simulink model "rollDynamicsLinear"  (R2017a)
settings: Solver=ode3  StartTime=0.0  StopTime=10  FixedStep=0.021  RelTol=1e-3  EnableMultiTasking=on
values from neighbouring files (symbols this model uses):
  enableMisErr = 1    [RollDynamics.m]    (also in RollDynamicsPWM-Theta.m = -1; rollDynamics.m)
  enableOutputPert = -1    [RollDynamics.m]    (also in RollDynamicsPWM-Theta.m)
  lambdaErr = 0.00001    (= 1e-05)    [RollDynamicsPWM-Theta.m]
  Mde = 70    [RollDynamicsPWM-Theta.m]
  Me = 15    [RollDynamicsPWM-Theta.m]
  roll_lin_den_84 = roll_lin_den_84{1,1}    [RollDynamicsPWM-Theta.m]
  roll_lin_num_84 = roll_lin_num_84{1,1}    [RollDynamicsPWM-Theta.m]
  Ts = 0.021    [RollDynamics.m]    (also in RollDynamicsPWM-Theta.m; rollDynamics.m)
undefined symbols (not defined in the file or in its folder): sigbuilder_block
libraries: simulink x7
settings Model: Creator=root  LastModifiedBy=userk
settings DataIOCC: LimitDataPoints=on  SaveFormat=Array
settings OptimizationCC: LifeSpan=inf
settings DebuggingCC: SolverPrmCheckMsg=warning  SFUnexpectedBacktrackingDiag=warning  SFNoUnconditionalDefaultTransitionDiag=warning  SFExecutionAtInitializationDiag=none
settings HardwareCC: ProdBitPerPointer=32  ProdBitPerSizeT=32  ProdBitPerPtrDiffT=32  ProdLargestAtomicFloat=None  ProdIntDivRoundTo=Undefined  ProdEndianess=Unspecified  ProdWordSize=32  ProdHWDeviceType=32-bit Generic
settings ModelReferenceCC: PropagateSignalLabelsOutOfModel=off
settings GRTTargetCC: TargetLangStandard=C89/C90 (ANSI)  GeneratePreprocessorConditionals=Disable all
settings ConfigComp: CovMetricSettings=dw  CovHtmlReporting=on  CovSaveCumulativeToWorkspaceVar=on  CovSaveSingleToWorkspaceVar=on  CovExternalEMLEnable=off  CovSFcnEnable=off

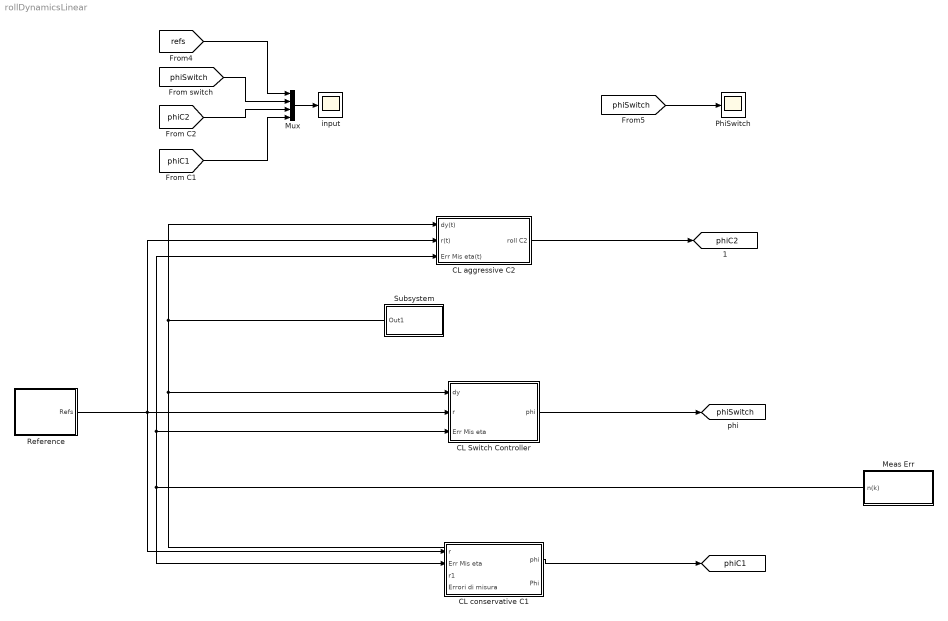
== system rollDynamicsLinear ==
  CL Switch Controller : Subsystem
  "CL aggressive C2 " : Subsystem
  CL conservative C1 : Subsystem
  Meas Err : Subsystem
  Mux : Mux
  PhiSwitch : Scope
  Reference : Subsystem
  Subsystem : Subsystem
  input : Scope
  tag scope: phiC1=global, phiC2=global, phiSwitch=global
  wires:
  Mux/1 -> input/1
  "CL aggressive C2 "/1(roll C2) -> [phiC2]
  CL conservative C1/1(phi) -> [phiC1]
  Reference/1(Refs) -> "CL aggressive C2 "/2(r(t)), CL Switch Controller/2(r), CL conservative C1/1(r)
  Subsystem/1(Out1) -> CL Switch Controller/1(dy), "CL aggressive C2 "/1(dy(t))
  Meas Err/1(n(k)) -> CL conservative C1/2(Err Mis eta), CL Switch Controller/3(Err Mis eta), "CL aggressive C2 "/3(Err Mis eta(t))
  CL Switch Controller/1(phi) -> [phiSwitch]
  [phiSwitch] -> Mux/2
  [phiC1] -> Mux/4
  [refs] -> Mux/1
  [phiSwitch] -> PhiSwitch/1
  [phiC2] -> Mux/3

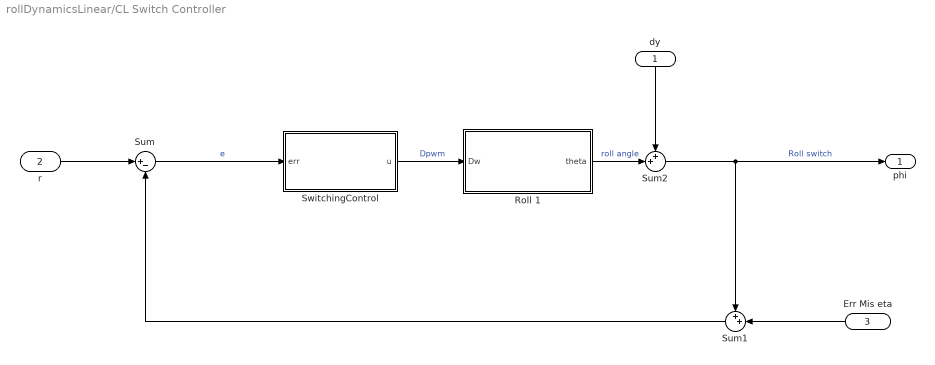
== system rollDynamicsLinear/CL Switch Controller ==
  dy : Inport
  r : Inport  Port=2
  Err Mis eta : Inport  Port=3
  Roll 1 : Subsystem
  Sum : Sum  Inputs=|+-
  Sum1 : Sum  Inputs=++|
  Sum2 : Sum  Inputs=++|
  "SwitchingControl " : Subsystem
  phi : Outport
  wires:
  r/1 -> Sum/1
  Sum2/1 -> phi/1, Sum1/1  "Roll switch"
  Roll 1/1("theta ") -> Sum2/2  "roll angle"
  "SwitchingControl "/1("u ") -> Roll 1/1("Dw ")  "Dpwm"
  Sum/1 -> "SwitchingControl "/1("err ")  "e"
  dy/1 -> Sum2/1
  Err Mis eta/1 -> Sum1/2
  Sum1/1 -> Sum/2

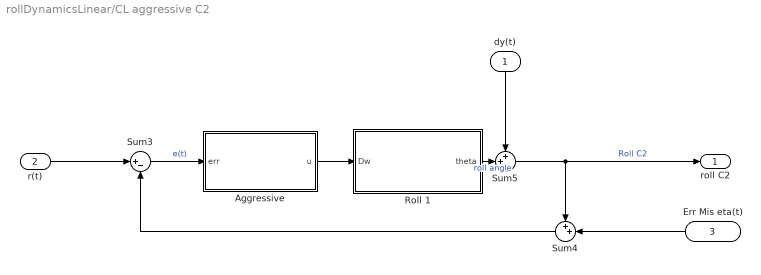
== system rollDynamicsLinear/CL aggressive C2  ==
  dy(t) : Inport
  r(t) : Inport  Port=2
  Err Mis eta(t) : Inport  Port=3
  "Aggressive " : Subsystem
  Roll 1 : Subsystem
  Sum3 : Sum  Inputs=|+-
  Sum4 : Sum  Inputs=++|
  Sum5 : Sum  Inputs=++|
  roll C2 : Outport
  wires:
  dy(t)/1 -> Sum5/1
  Sum3/1 -> "Aggressive "/1("err ")  "e(t)"
  "Aggressive "/1("u ") -> Roll 1/1("Dw ")
  Sum4/1 -> Sum3/2
  Sum5/1 -> roll C2/1, Sum4/1  "Roll C2"
  r(t)/1 -> Sum3/1
  Roll 1/1("theta ") -> Sum5/2  "roll angle"
  Err Mis eta(t)/1 -> Sum4/2

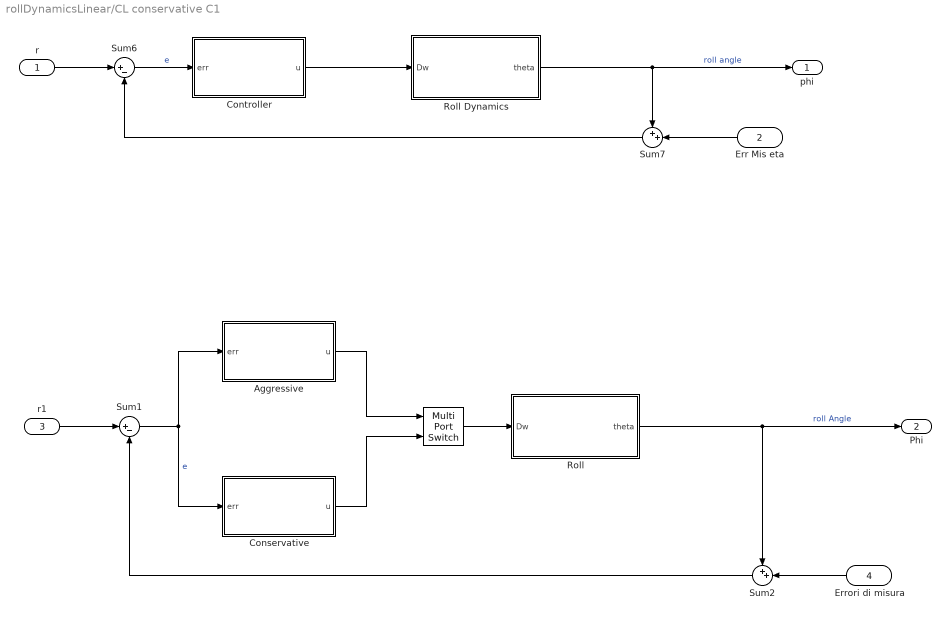
== system rollDynamicsLinear/CL conservative C1 ==
  r : Inport
  Err Mis eta : Inport  Port=2
  r1 : Inport  Port=3
  Errori di misura : Inport  Port=4
  " " : MultiPortSwitch  DataPortOrder=Zero-based contiguous  Inputs=1  zeroidx=on
  "Aggressive " : Subsystem
  Conservative : Subsystem
  Controller : Subsystem
  "Roll " : Subsystem
  "Roll Dynamics " : Subsystem
  Sum1 : Sum  Inputs=|+-
  Sum2 : Sum  Inputs=++|
  Sum6 : Sum  Inputs=|+-
  Sum7 : Sum  Inputs=++|
  phi : Outport
  Phi : Outport  Port=2
  wires:
  Err Mis eta/1 -> Sum7/2
  r/1 -> Sum6/1
  "Roll Dynamics "/1("theta ") -> phi/1, Sum7/1  "roll angle"
  Sum6/1 -> Controller/1("err ")  "e"
  Sum7/1 -> Sum6/2
  Controller/1("u ") -> "Roll Dynamics "/1("Dw ")
  Errori di misura/1 -> Sum2/2
  "Roll "/1("theta ") -> Phi/1, Sum2/1  "roll Angle"
  Sum1/1 -> Conservative/1("err "), "Aggressive "/1("err ")  "e"
  Sum2/1 -> Sum1/2
  r1/1 -> Sum1/1
  Conservative/1("u ") -> " "/2
  " "/1 -> "Roll "/1("Dw ")
  "Aggressive "/1("u ") -> " "/1

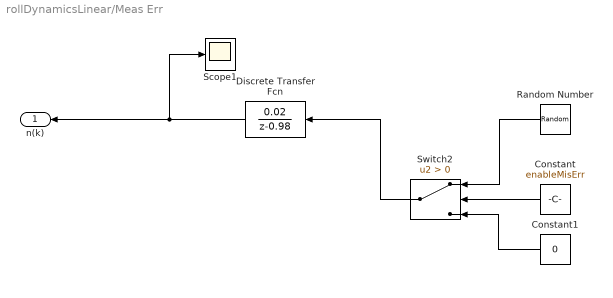
== system rollDynamicsLinear/Meas Err ==
  Constant : Constant  Value=enableMisErr
  Constant1 : Constant  Value=0
  Discrete Transfer Fcn : DiscreteTransferFcn  Numerator=[0.02]  Denominator=[1 -0.98]
  Random Number : RandomNumber  Variance=1.3  SampleTime=Ts
  Scope1 : Scope
  Switch2 : Switch  Criteria=u2 > Threshold  SampleTime=Ts
  n(k) : Outport
  wires:
  Constant1/1 -> Switch2/3
  Constant/1 -> Switch2/2
  Random Number/1 -> Switch2/1
  Switch2/1 -> Discrete Transfer Fcn/1
  Discrete Transfer Fcn/1 -> Scope1/1, n(k)/1

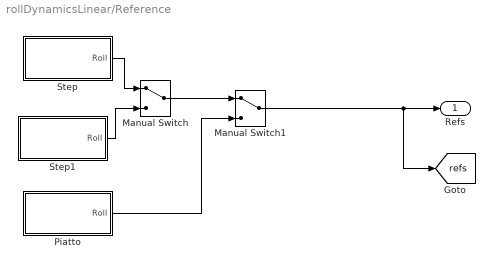
== system rollDynamicsLinear/Reference ==
  Manual Switch : ManualSwitch
  Manual Switch1 : ManualSwitch
  Piatto : Subsystem  Tag=STV Subsys  LoadFcn=sigbuilder_block('load');  StartFcn=sigbuilder_block('start');  StopFcn=sigbuilder_block('stop');  ClipboardFcn=sigbuilder_block('clipboard');  mask(Sigbuilder block){tuvar=[0:10]}
      mask help: Simulink:masks:SigbuilderBlock_MD
      mask init:
      | if ~strcmp(get_param(bdroot(gcbh),'SimulationStatus'),'stopped') tuvar = sigbuilder_block('maskInit'); end
      settings: CopyFcn=sigbuilder_block('copy');  DeleteFcn=sigbuilder_block('delete');  ModelCloseFcn=sigbuilder_block('modelClose');  PreSaveFcn=sigbuilder_block('preSave');  PauseFcn=sigbuilder_block('pause');  ContinueFcn=sigbuilder_block('continue');  NameChangeFcn=sigbuilder_block('namechange');  OpenFcn=sigbuilder_block('open',[240 0.75 594.75 533.25 ]);  CloseFcn=sigbuilder_block('close');
      mask Display: plot(0, 0, 100, 100,[2, 2, 32, 32, 2], [68, 8, 8, 68, 68],[32, 2], [38, 38], [32, 19, 2],[53, 60, 44], [32, 17, 17, 2],[16, 16, 31, 31]);txt = getActiveGroup(gcbh);text(2, 100, txt,'verticalAlignment', 'top');
  Step : Subsystem  Tag=STV Subsys  LoadFcn=sigbuilder_block('load');  StartFcn=sigbuilder_block('start');  StopFcn=sigbuilder_block('stop');  ClipboardFcn=sigbuilder_block('clipboard');  mask(Sigbuilder block){tuvar=[0:10]}
      mask help: Simulink:masks:SigbuilderBlock_MD
      mask init:
      | if ~strcmp(get_param(bdroot(gcbh),'SimulationStatus'),'stopped') tuvar = sigbuilder_block('maskInit'); end
      settings: CopyFcn=sigbuilder_block('copy');  DeleteFcn=sigbuilder_block('delete');  ModelCloseFcn=sigbuilder_block('modelClose');  PreSaveFcn=sigbuilder_block('preSave');  PauseFcn=sigbuilder_block('pause');  ContinueFcn=sigbuilder_block('continue');  NameChangeFcn=sigbuilder_block('namechange');  OpenFcn=sigbuilder_block('open',[222.75 0 632.25 495.75 ]);  CloseFcn=sigbuilder_block('close');
      mask Display: plot(0, 0, 100, 100,[2, 2, 32, 32, 2], [68, 8, 8, 68, 68],[32, 2], [38, 38], [32, 19, 2],[53, 60, 44], [32, 17, 17, 2],[16, 16, 31, 31]);txt = getActiveGroup(gcbh);text(2, 100, txt,'verticalAlignment', 'top');
  Step1 : Subsystem  Tag=STV Subsys  LoadFcn=sigbuilder_block('load');  StartFcn=sigbuilder_block('start');  StopFcn=sigbuilder_block('stop');  ClipboardFcn=sigbuilder_block('clipboard');  mask(Sigbuilder block){tuvar=[0:10]}
      mask help: Simulink:masks:SigbuilderBlock_MD
      mask init:
      | if ~strcmp(get_param(bdroot(gcbh),'SimulationStatus'),'stopped') tuvar = sigbuilder_block('maskInit'); end
      settings: CopyFcn=sigbuilder_block('copy');  DeleteFcn=sigbuilder_block('delete');  ModelCloseFcn=sigbuilder_block('modelClose');  PreSaveFcn=sigbuilder_block('preSave');  PauseFcn=sigbuilder_block('pause');  ContinueFcn=sigbuilder_block('continue');  NameChangeFcn=sigbuilder_block('namechange');  OpenFcn=sigbuilder_block('open',[222.75 0 632.25 495.75 ]);  CloseFcn=sigbuilder_block('close');
      mask Display: plot(0, 0, 100, 100,[2, 2, 32, 32, 2], [68, 8, 8, 68, 68],[32, 2], [38, 38], [32, 19, 2],[53, 60, 44], [32, 17, 17, 2],[16, 16, 31, 31]);txt = getActiveGroup(gcbh);text(2, 100, txt,'verticalAlignment', 'top');
  Refs : Outport
  tag scope: refs=global
  wires:
  Step/1(Roll) -> Manual Switch/1
  Step1/1(Roll) -> Manual Switch/2
  Manual Switch/1 -> Manual Switch1/1
  Piatto/1(Roll) -> Manual Switch1/2
  Manual Switch1/1 -> [refs], Refs/1

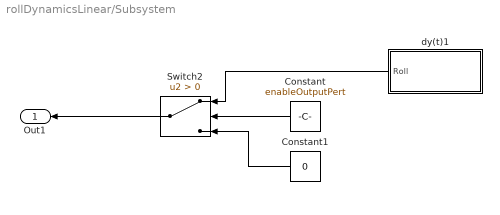
== system rollDynamicsLinear/Subsystem ==
  Constant : Constant  Value=enableOutputPert  SampleTime=Ts
  Constant1 : Constant  Value=0
  Switch2 : Switch  Criteria=u2 > Threshold  SampleTime=Ts
  dy(t)1 : Subsystem  Tag=STV Subsys  LoadFcn=sigbuilder_block('load');  StartFcn=sigbuilder_block('start');  StopFcn=sigbuilder_block('stop');  ClipboardFcn=sigbuilder_block('clipboard');  mask(Sigbuilder block){tuvar=[0:10]}
      mask help: Simulink:masks:SigbuilderBlock_MD
      mask init:
      | if ~strcmp(get_param(bdroot(gcbh),'SimulationStatus'),'stopped') tuvar = sigbuilder_block('maskInit'); end
      settings: CopyFcn=sigbuilder_block('copy');  DeleteFcn=sigbuilder_block('delete');  ModelCloseFcn=sigbuilder_block('modelClose');  PreSaveFcn=sigbuilder_block('preSave');  PauseFcn=sigbuilder_block('pause');  ContinueFcn=sigbuilder_block('continue');  NameChangeFcn=sigbuilder_block('namechange');  OpenFcn=sigbuilder_block('open',[234.75 0 602.25 495.75 ]);  CloseFcn=sigbuilder_block('close');
      mask Display: plot(0, 0, 100, 100,[2, 2, 32, 32, 2], [68, 8, 8, 68, 68],[32, 2], [38, 38], [32, 19, 2],[53, 60, 44], [32, 17, 17, 2],[16, 16, 31, 31]);txt = getActiveGroup(gcbh);text(2, 100, txt,'verticalAlignment', 'top');
  Out1 : Outport
  wires:
  Constant1/1 -> Switch2/3
  Constant/1 -> Switch2/2
  Switch2/1 -> Out1/1
  dy(t)1/1(Roll) -> Switch2/1

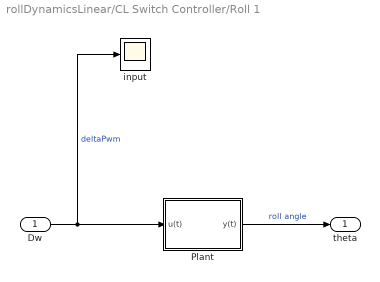
== system rollDynamicsLinear/CL Switch Controller/Roll 1 ==
  "Dw " : Inport
  Plant : Subsystem
  input : Scope
  "theta " : Outport
  wires:
  Plant/1(y(t)) -> "theta "/1  "roll angle"
  "Dw "/1 -> Plant/1(u(t)), input/1  "deltaPwm"

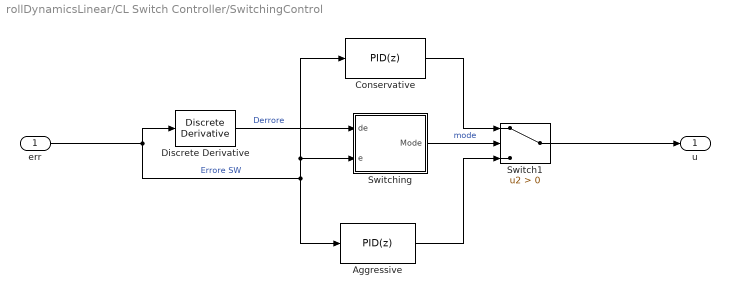
== system rollDynamicsLinear/CL Switch Controller/SwitchingControl  ==
  "err " : Inport
  Aggressive : simulink/Continuous/PID Controller  Controller=PID  TimeDomain=Discrete-time  SampleTime=Ts  IntegratorMethod=Forward Euler  FilterMethod=Forward Euler  Form=Parallel  UseFilter=on  ControllerParametersSource=internal  P=4.42475572373396  I=4.1750628142498  D=1.09206142677048  N=72.8133379098477  InitialConditionSource=internal  InitialConditionForIntegrator=0  InitialConditionForFilter=0  ExternalReset=none  LimitOutput=off  UpperSaturationLimit=inf  LowerSaturationLimit=-inf  LinearizeAsGain=off  AntiWindupMode=none  Kb=1  TrackingMode=off  Kt=1  PParamMin=[]  PParamMax=[]  IParamMin=[]  IParamMax=[]  DParamMin=[]  DParamMax=[]  NParamMin=[]  NParamMax=[]  KbParamMin=[]  KbParamMax=[]  KtParamMin=[]  KtParamMax=[]  POutMin=[]  POutMax=[]  IOutMin=[]  IOutMax=[]  DOutMin=[]  DOutMax=[]  NOutMin=[]  NOutMax=[]  KbOutMin=[]  KbOutMax=[]  KtOutMin=[]  KtOutMax=[]  IntegratorOutMin=[]  IntegratorOutMax=[]  FilterOutMin=[]  FilterOutMax=[]  SumOutMin=[]  SumOutMax=[]  SumI1OutMin=[]  SumI1OutMax=[]  SumI2OutMin=[]  SumI2OutMax=[]  SumI3OutMin=[]  SumI3OutMax=[]  SumDOutMin=[]  SumDOutMax=[]  SaturationOutMin=[]  SaturationOutMax=[]  IntegratorContinuousStateAttributes=''  IntegratorStateMustResolveToSignalObject=off  IntegratorRTWStateStorageClass=Auto  FilterContinuousStateAttributes=''  FilterStateMustResolveToSignalObject=off  FilterRTWStateStorageClass=Auto  DifferentiatorICPrevScaledInput=0  DifferentiatorOutMin=[]  DifferentiatorOutMax=[]  InitialConditionSetting=State (most efficient)
  Conservative : simulink/Continuous/PID Controller  Controller=PID  TimeDomain=Discrete-time  SampleTime=Ts  IntegratorMethod=Forward Euler  FilterMethod=Forward Euler  Form=Parallel  UseFilter=off  ControllerParametersSource=internal  P=12.3804823161569  I=9.71645786209043  D=3.69266333876468  N=74.1578480478725  InitialConditionSource=internal  InitialConditionForIntegrator=0  InitialConditionForFilter=0  ExternalReset=none  LimitOutput=off  UpperSaturationLimit=inf  LowerSaturationLimit=-inf  LinearizeAsGain=off  AntiWindupMode=none  Kb=1  TrackingMode=off  Kt=1  PParamMin=[]  PParamMax=[]  IParamMin=[]  IParamMax=[]  DParamMin=[]  DParamMax=[]  NParamMin=[]  NParamMax=[]  KbParamMin=[]  KbParamMax=[]  KtParamMin=[]  KtParamMax=[]  POutMin=[]  POutMax=[]  IOutMin=[]  IOutMax=[]  DOutMin=[]  DOutMax=[]  NOutMin=[]  NOutMax=[]  KbOutMin=[]  KbOutMax=[]  KtOutMin=[]  KtOutMax=[]  IntegratorOutMin=[]  IntegratorOutMax=[]  FilterOutMin=[]  FilterOutMax=[]  SumOutMin=[]  SumOutMax=[]  SumI1OutMin=[]  SumI1OutMax=[]  SumI2OutMin=[]  SumI2OutMax=[]  SumI3OutMin=[]  SumI3OutMax=[]  SumDOutMin=[]  SumDOutMax=[]  SaturationOutMin=[]  SaturationOutMax=[]  IntegratorContinuousStateAttributes=''  IntegratorStateMustResolveToSignalObject=off  IntegratorRTWStateStorageClass=Auto  FilterContinuousStateAttributes=''  FilterStateMustResolveToSignalObject=off  FilterRTWStateStorageClass=Auto  DifferentiatorICPrevScaledInput=0  DifferentiatorOutMin=[]  DifferentiatorOutMax=[]  InitialConditionSetting=State (most efficient)
  Discrete Derivative : simulink/Discrete/Discrete Derivative  gainval=1.0  ICPrevScaledInput=0.0  OutMin=[]  OutMax=[]  OutDataType=fixdt(1, 16)  OutScaling=2^-10  DoSatur=off
  Switch1 : Switch  Criteria=u2 > Threshold
  Switching : Subsystem
  "u " : Outport
  wires:
  Aggressive/1 -> Switch1/3
  Conservative/1 -> Switch1/1
  "err "/1 -> Discrete Derivative/1, Aggressive/1, Conservative/1, Switching/2(e)  "Errore SW"
  Discrete Derivative/1 -> Switching/1(de)  "Derrore"
  Switching/1(Mode) -> Switch1/2  "mode"
  Switch1/1 -> "u "/1

== system rollDynamicsLinear/CL aggressive C2 /Aggressive  ==
  "err " : Inport
  Aggressive : simulink/Continuous/PID Controller  Controller=PID  TimeDomain=Discrete-time  SampleTime=Ts  IntegratorMethod=Forward Euler  FilterMethod=Forward Euler  Form=Parallel  UseFilter=on  ControllerParametersSource=internal  P=4.42475572373396  I=4.1750628142498  D=1.09206142677048  N=72.8133379098477  InitialConditionSource=internal  InitialConditionForIntegrator=0  InitialConditionForFilter=0  ExternalReset=none  LimitOutput=off  UpperSaturationLimit=inf  LowerSaturationLimit=-inf  LinearizeAsGain=off  AntiWindupMode=none  Kb=1  TrackingMode=off  Kt=1  PParamMin=[]  PParamMax=[]  IParamMin=[]  IParamMax=[]  DParamMin=[]  DParamMax=[]  NParamMin=[]  NParamMax=[]  KbParamMin=[]  KbParamMax=[]  KtParamMin=[]  KtParamMax=[]  POutMin=[]  POutMax=[]  IOutMin=[]  IOutMax=[]  DOutMin=[]  DOutMax=[]  NOutMin=[]  NOutMax=[]  KbOutMin=[]  KbOutMax=[]  KtOutMin=[]  KtOutMax=[]  IntegratorOutMin=[]  IntegratorOutMax=[]  FilterOutMin=[]  FilterOutMax=[]  SumOutMin=[]  SumOutMax=[]  SumI1OutMin=[]  SumI1OutMax=[]  SumI2OutMin=[]  SumI2OutMax=[]  SumI3OutMin=[]  SumI3OutMax=[]  SumDOutMin=[]  SumDOutMax=[]  SaturationOutMin=[]  SaturationOutMax=[]  IntegratorContinuousStateAttributes=''  IntegratorStateMustResolveToSignalObject=off  IntegratorRTWStateStorageClass=Auto  FilterContinuousStateAttributes=''  FilterStateMustResolveToSignalObject=off  FilterRTWStateStorageClass=Auto  DifferentiatorICPrevScaledInput=0  DifferentiatorOutMin=[]  DifferentiatorOutMax=[]  InitialConditionSetting=State (most efficient)
  "u " : Outport
  wires:
  "err "/1 -> Aggressive/1  "Err Agg"
  Aggressive/1 -> "u "/1

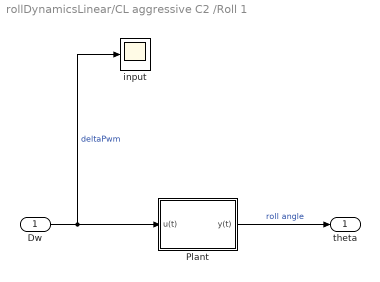
== system rollDynamicsLinear/CL aggressive C2 /Roll 1 ==
  "Dw " : Inport
  Plant : Subsystem
  input : Scope
  "theta " : Outport
  wires:
  Plant/1(y(t)) -> "theta "/1  "roll angle"
  "Dw "/1 -> Plant/1(u(t)), input/1  "deltaPwm"

== system rollDynamicsLinear/CL conservative C1/Aggressive  ==
  "err " : Inport
  Aggressive : simulink/Continuous/PID Controller  Controller=PID  TimeDomain=Discrete-time  SampleTime=Ts  IntegratorMethod=Forward Euler  FilterMethod=Forward Euler  Form=Parallel  UseFilter=on  ControllerParametersSource=internal  P=4.42475572373396  I=4.1750628142498  D=1.09206142677048  N=72.8133379098477  InitialConditionSource=internal  InitialConditionForIntegrator=0  InitialConditionForFilter=0  ExternalReset=none  LimitOutput=off  UpperSaturationLimit=inf  LowerSaturationLimit=-inf  LinearizeAsGain=off  AntiWindupMode=none  Kb=1  TrackingMode=off  Kt=1  PParamMin=[]  PParamMax=[]  IParamMin=[]  IParamMax=[]  DParamMin=[]  DParamMax=[]  NParamMin=[]  NParamMax=[]  KbParamMin=[]  KbParamMax=[]  KtParamMin=[]  KtParamMax=[]  POutMin=[]  POutMax=[]  IOutMin=[]  IOutMax=[]  DOutMin=[]  DOutMax=[]  NOutMin=[]  NOutMax=[]  KbOutMin=[]  KbOutMax=[]  KtOutMin=[]  KtOutMax=[]  IntegratorOutMin=[]  IntegratorOutMax=[]  FilterOutMin=[]  FilterOutMax=[]  SumOutMin=[]  SumOutMax=[]  SumI1OutMin=[]  SumI1OutMax=[]  SumI2OutMin=[]  SumI2OutMax=[]  SumI3OutMin=[]  SumI3OutMax=[]  SumDOutMin=[]  SumDOutMax=[]  SaturationOutMin=[]  SaturationOutMax=[]  IntegratorContinuousStateAttributes=''  IntegratorStateMustResolveToSignalObject=off  IntegratorRTWStateStorageClass=Auto  FilterContinuousStateAttributes=''  FilterStateMustResolveToSignalObject=off  FilterRTWStateStorageClass=Auto  DifferentiatorICPrevScaledInput=0  DifferentiatorOutMin=[]  DifferentiatorOutMax=[]  InitialConditionSetting=State (most efficient)
  "u " : Outport
  wires:
  "err "/1 -> Aggressive/1  "Err Agg"
  Aggressive/1 -> "u "/1

== system rollDynamicsLinear/CL conservative C1/Conservative ==
  "err " : Inport
  Conservative : simulink/Continuous/PID Controller  Controller=PID  TimeDomain=Discrete-time  SampleTime=Ts  IntegratorMethod=Forward Euler  FilterMethod=Forward Euler  Form=Parallel  UseFilter=off  ControllerParametersSource=internal  P=12.3804823161569  I=9.71645786209043  D=3.69266333876468  N=74.1578480478725  InitialConditionSource=internal  InitialConditionForIntegrator=0  InitialConditionForFilter=0  ExternalReset=none  LimitOutput=off  UpperSaturationLimit=inf  LowerSaturationLimit=-inf  LinearizeAsGain=off  AntiWindupMode=none  Kb=1  TrackingMode=off  Kt=1  PParamMin=[]  PParamMax=[]  IParamMin=[]  IParamMax=[]  DParamMin=[]  DParamMax=[]  NParamMin=[]  NParamMax=[]  KbParamMin=[]  KbParamMax=[]  KtParamMin=[]  KtParamMax=[]  POutMin=[]  POutMax=[]  IOutMin=[]  IOutMax=[]  DOutMin=[]  DOutMax=[]  NOutMin=[]  NOutMax=[]  KbOutMin=[]  KbOutMax=[]  KtOutMin=[]  KtOutMax=[]  IntegratorOutMin=[]  IntegratorOutMax=[]  FilterOutMin=[]  FilterOutMax=[]  SumOutMin=[]  SumOutMax=[]  SumI1OutMin=[]  SumI1OutMax=[]  SumI2OutMin=[]  SumI2OutMax=[]  SumI3OutMin=[]  SumI3OutMax=[]  SumDOutMin=[]  SumDOutMax=[]  SaturationOutMin=[]  SaturationOutMax=[]  IntegratorContinuousStateAttributes=''  IntegratorStateMustResolveToSignalObject=off  IntegratorRTWStateStorageClass=Auto  FilterContinuousStateAttributes=''  FilterStateMustResolveToSignalObject=off  FilterRTWStateStorageClass=Auto  DifferentiatorICPrevScaledInput=0  DifferentiatorOutMin=[]  DifferentiatorOutMax=[]  InitialConditionSetting=State (most efficient)
  "u " : Outport
  wires:
  "err "/1 -> Conservative/1  "Err Cons"
  Conservative/1 -> "u "/1

== system rollDynamicsLinear/CL conservative C1/Controller ==
  "err " : Inport
  Conservative : simulink/Continuous/PID Controller  Controller=PID  TimeDomain=Discrete-time  SampleTime=Ts  IntegratorMethod=Forward Euler  FilterMethod=Forward Euler  Form=Parallel  UseFilter=off  ControllerParametersSource=internal  P=12.3804823161569  I=9.71645786209043  D=3.69266333876468  N=74.1578480478725  InitialConditionSource=internal  InitialConditionForIntegrator=0  InitialConditionForFilter=0  ExternalReset=none  LimitOutput=off  UpperSaturationLimit=inf  LowerSaturationLimit=-inf  LinearizeAsGain=off  AntiWindupMode=none  Kb=1  TrackingMode=off  Kt=1  PParamMin=[]  PParamMax=[]  IParamMin=[]  IParamMax=[]  DParamMin=[]  DParamMax=[]  NParamMin=[]  NParamMax=[]  KbParamMin=[]  KbParamMax=[]  KtParamMin=[]  KtParamMax=[]  POutMin=[]  POutMax=[]  IOutMin=[]  IOutMax=[]  DOutMin=[]  DOutMax=[]  NOutMin=[]  NOutMax=[]  KbOutMin=[]  KbOutMax=[]  KtOutMin=[]  KtOutMax=[]  IntegratorOutMin=[]  IntegratorOutMax=[]  FilterOutMin=[]  FilterOutMax=[]  SumOutMin=[]  SumOutMax=[]  SumI1OutMin=[]  SumI1OutMax=[]  SumI2OutMin=[]  SumI2OutMax=[]  SumI3OutMin=[]  SumI3OutMax=[]  SumDOutMin=[]  SumDOutMax=[]  SaturationOutMin=[]  SaturationOutMax=[]  IntegratorContinuousStateAttributes=''  IntegratorStateMustResolveToSignalObject=off  IntegratorRTWStateStorageClass=Auto  FilterContinuousStateAttributes=''  FilterStateMustResolveToSignalObject=off  FilterRTWStateStorageClass=Auto  DifferentiatorICPrevScaledInput=0  DifferentiatorOutMin=[]  DifferentiatorOutMax=[]  InitialConditionSetting=State (most efficient)
  "u " : Outport
  wires:
  "err "/1 -> Conservative/1  "Err Cons"
  Conservative/1 -> "u "/1

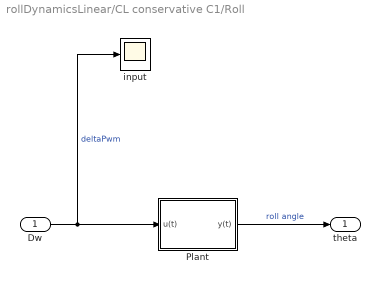
== system rollDynamicsLinear/CL conservative C1/Roll  ==
  "Dw " : Inport
  Plant : Subsystem
  input : Scope
  "theta " : Outport
  wires:
  Plant/1(y(t)) -> "theta "/1  "roll angle"
  "Dw "/1 -> Plant/1(u(t)), input/1  "deltaPwm"

== system rollDynamicsLinear/CL conservative C1/Roll Dynamics  ==
  "Dw " : Inport
  Plant : Subsystem
  input : Scope
  "theta " : Outport
  wires:
  Plant/1(y(t)) -> "theta "/1  "roll angle"
  "Dw "/1 -> Plant/1(u(t)), input/1  "deltaPwm"

== system rollDynamicsLinear/Reference/Piatto ==
  Demux : Demux  Tag=STV Demux  Outputs=1
  FromWs : FromWorkspace  Tag=STV FromWs  VariableName=tuvar  SampleTime=0
      SigBuilderData=|
      | common.afterFinalStr = 'Extrapolate'
      | common.sampleTime = 0
      | dataSet.timeRange = [0 10]
      | dataSet.name = 'Group 1'
      | sbobj.Groups.Name = 'Group 1'
      | sbobj.Groups.Signals.Name = 'Roll'
      | sbobj.Groups.Signals.XData = [0 10]
      | sbobj.Groups.Signals.YData = [0 0]
  Roll : Outport  Tag=STV Outport
  wires:
  FromWs/1 -> Demux/1
  Demux/1 -> Roll/1

== system rollDynamicsLinear/Reference/Step ==
  Demux : Demux  Tag=STV Demux  Outputs=1
  FromWs : FromWorkspace  Tag=STV FromWs  VariableName=tuvar  SampleTime=Ts
      SigBuilderData=|
      | common.afterFinalStr = 'Extrapolate'
      | common.sampleTime = 'Ts'
      | dataSet.timeRange = [0 20]
      | dataSet.name = 'Group 1'
      | sbobj.Groups.Name = 'Group 1'
      | sbobj.Groups.Signals.Name = 'Roll'
      | sbobj.Groups.Signals.XData = [0 2 2 10.1 20]
      | sbobj.Groups.Signals.YData = [0 0 10 10 10]
      | sbobj.Groups.TimeRange = [0 20]
  Roll : Outport  Tag=STV Outport
  wires:
  FromWs/1 -> Demux/1
  Demux/1 -> Roll/1

== system rollDynamicsLinear/Reference/Step1 ==
  Demux : Demux  Tag=STV Demux  Outputs=1
  FromWs : FromWorkspace  Tag=STV FromWs  VariableName=tuvar  SampleTime=Ts
      SigBuilderData=|
      | common.afterFinalStr = 'Extrapolate'
      | common.sampleTime = 'Ts'
      | dataSet.timeRange = [0 20]
      | dataSet.name = 'Group 1'
      | sbobj.Groups.Name = 'Group 1'
      | sbobj.Groups.Signals.Name = 'Roll'
      | sbobj.Groups.Signals.XData = [0 2 2 10.1 10.1 20]
      | sbobj.Groups.Signals.YData = [0 0 10 10 0 0]
      | sbobj.Groups.TimeRange = [0 20]
  Roll : Outport  Tag=STV Outport
  wires:
  FromWs/1 -> Demux/1
  Demux/1 -> Roll/1

== system rollDynamicsLinear/Subsystem/dy(t)1 ==
  Demux : Demux  Tag=STV Demux  Outputs=1
  FromWs : FromWorkspace  Tag=STV FromWs  VariableName=tuvar  SampleTime=0
      SigBuilderData=|
      | common.afterFinalStr = 'Extrapolate'
      | common.sampleTime = 0
      | dataSet.timeRange = [0 10]
      | dataSet.name = 'Group 1'
      | sbobj.Groups.Name = 'Group 1'
      | sbobj.Groups.Signals.Name = 'Roll'
      | sbobj.Groups.Signals.XData = [0 4 4 4.06 4.06 10]
      | sbobj.Groups.Signals.YData = [0 0 20 20 0 0]
  Roll : Outport  Tag=STV Outport
  wires:
  Demux/1 -> Roll/1
  FromWs/1 -> Demux/1

== system rollDynamicsLinear/CL Switch Controller/Roll 1/Plant ==
  u(t) : Inport
  P(s) : DiscreteTransferFcn  Numerator=roll_lin_num_84  Denominator=roll_lin_den_84  SampleTime=Ts
  y(t) : Outport
  wires:
  P(s)/1 -> y(t)/1
  u(t)/1 -> P(s)/1

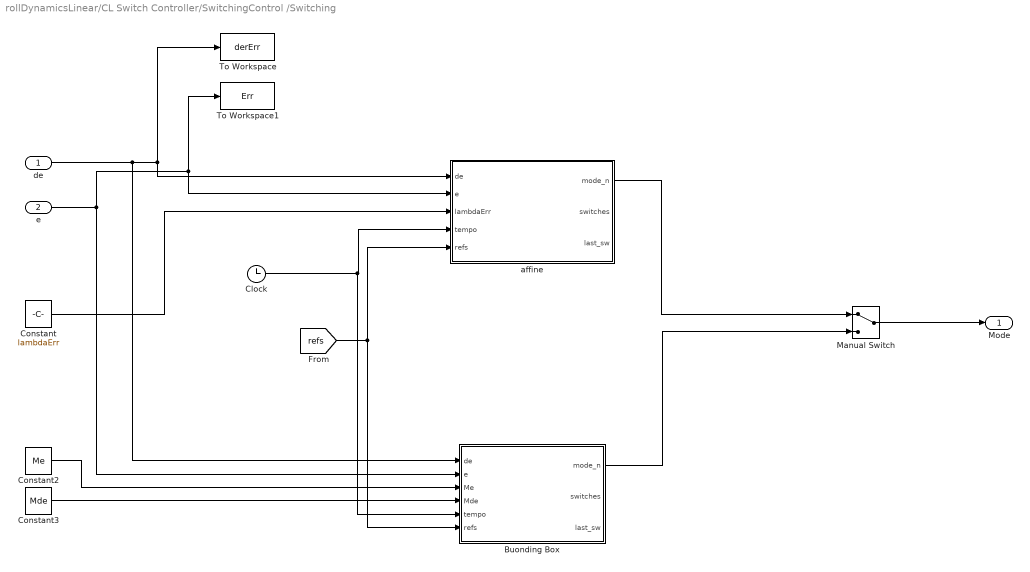
== system rollDynamicsLinear/CL Switch Controller/SwitchingControl /Switching ==
  de : Inport
  e : Inport  Port=2
  Buonding Box : MATLAB Function  TreatAsAtomicUnit=on
  Clock : Clock
  Constant : Constant  Value=lambdaErr
  Constant2 : Constant  Value=Me
  Constant3 : Constant  Value=Mde
  Manual Switch : ManualSwitch
  To Workspace : ToWorkspace  VariableName=derErr  SaveFormat=Timeseries  SampleTime=-1
  To Workspace1 : ToWorkspace  VariableName=Err  SaveFormat=Timeseries  SampleTime=-1
  affine : MATLAB Function  TreatAsAtomicUnit=on
  Mode : Outport
  wires:
  Constant/1 -> affine/3(lambdaErr)
  e/1 -> Buonding Box/2(e), To Workspace1/1, affine/2(e)
  de/1 -> Buonding Box/1(de), To Workspace/1, affine/1(de)
  Manual Switch/1 -> Mode/1
  affine/1(mode_n) -> Manual Switch/1
  Buonding Box/1(mode_n) -> Manual Switch/2
  Constant3/1 -> Buonding Box/4(Mde)
  Constant2/1 -> Buonding Box/3(Me)
  Clock/1 -> Buonding Box/5(tempo), affine/4(tempo)
  [refs] -> Buonding Box/6(refs), affine/5(refs)

== system rollDynamicsLinear/CL aggressive C2 /Roll 1/Plant ==
  u(t) : Inport
  P(s) : DiscreteTransferFcn  Numerator=roll_lin_num_84  Denominator=roll_lin_den_84  SampleTime=Ts
  y(t) : Outport
  wires:
  P(s)/1 -> y(t)/1
  u(t)/1 -> P(s)/1

== system rollDynamicsLinear/CL conservative C1/Roll /Plant ==
  u(t) : Inport
  P(s) : DiscreteTransferFcn  Numerator=roll_lin_num_84  Denominator=roll_lin_den_84  SampleTime=Ts
  y(t) : Outport
  wires:
  P(s)/1 -> y(t)/1
  u(t)/1 -> P(s)/1

== system rollDynamicsLinear/CL conservative C1/Roll Dynamics /Plant ==
  u(t) : Inport
  P(s) : DiscreteTransferFcn  Numerator=roll_lin_num_84  Denominator=roll_lin_den_84  SampleTime=Ts
  y(t) : Outport
  wires:
  P(s)/1 -> y(t)/1
  u(t)/1 -> P(s)/1

== matlab function rollDynamicsLinear/CL Switch Controller/SwitchingControl /Switching/affine ==
  data: de input; e input; mode_n output; lambdaErr input; tempo input; refs input; switches output; last_sw output
function [mode_n,switches,last_sw] = checkCondE(de,e,lambdaErr,tempo,refs)
%#codegen
persistent last_switch mode_m1 num_switch ref_m1 max_switch mode


if isempty(mode) 
    mode = 1;
end

if isempty(mode_m1) 
    mode_m1 = mode;
end

if isempty(num_switch)
    num_switch = 0;
end
if isempty(last_switch) 
    last_switch = tempo;
end

if isempty(ref_m1) 
    ref_m1 = refs;
end

if isempty(max_switch) 
    max_switch = 0;
end

if abs(refs - ref_m1) > 0
    max_switch = 2;
    num_switch = 0;
end

dwell_time = 0.9;

if tempo - last_switch >= dwell_time && num_switch < max_switch 
    if de ~= 0 && e ~= 0
        if de > 0 && e > 0
            % primo quadrante
            if de - lambdaErr/e <= 0
            %if de <= 20 && e <= 6
                 mode = 1;
                 if mode_m1 == -1
                   last_switch = tempo;
                   num_switch = num_switch + 1;
                 end

            else
                mode = -1;
                if mode_m1 == 1
                   last_switch = tempo;
                   num_switch = num_switch + 1;
                end
            end
        elseif de < 0 && e > 0
            % second quadrante
            if de + lambdaErr/e <= 0
            %if de >= -25 && e <= 5
                 mode = 1;
                if mode_m1 == -1
                   last_switch = tempo
                   num_switch = num_switch + 1;
                end
            else
                mode = -1;
                if mode_m1 == 1
                   last_switch = tempo;
                   num_switch = num_switch + 1;
                end
            end
        elseif de > 0 && e < 0
            % quarto quadrante
            if de + lambdaErr/e <= 0
                 mode = 1;
                if mode_m1 == -1
                   last_switch = tempo;
                   num_switch = num_switch + 1;
                end
            else
                mode = -1;
                if mode_m1 == 1
                   last_switch = tempo;
                   num_switch = num_switch + 1;
                end
            end
        elseif de < 0 && e < 0
            % terzo quadrante
            if de + lambdaErr/(-e) <= 0
                 mode = 1;
                if mode_m1 == -1
                   last_switch = tempo;
                   num_switch = num_switch + 1;
                end
            else
                mode = -1;
                if mode_m1 == 1
                   last_switch = tempo;
                   num_switch = num_switch + 1;
                end
            end
        end
    end
end

mode_m1 = mode;
ref_m1 = refs;
switches = num_switch;
last_sw = last_switch;
mode_n = mode;
    
end

== matlab function rollDynamicsLinear/CL Switch Controller/SwitchingControl /Switching/Buonding Box ==
  data: de input; e input; mode_n output; Me input; Mde input; tempo input; refs input; switches output; last_sw output
function [mode_n,switches,last_sw]= checkCondE(de,e,Me,Mde,tempo,refs)
%#codegen
persistent last_switch mode_m1 num_switch ref_m1 max_switch mode


if isempty(mode_m1) 
    mode_m1 = -1;
end
if isempty(num_switch)
    num_switch = 0;
end
if isempty(last_switch) 
    last_switch = tempo;
end

if isempty(ref_m1) 
    ref_m1 = refs;
end

if isempty(mode) 
    mode = -1;
end

if isempty(max_switch) 
    max_switch = 0;
end

if abs(refs - ref_m1) > 0
    max_switch = 5;
    num_switch = 0;
end

dwell_time = 0.01;

if tempo - last_switch >= dwell_time && num_switch < max_switch  
    if de ~= 0 && e ~= 0
        if de >= 0 && e >= 0
            % primo quadrante
            if de <= Mde && e <= Me
                 mode = 1;
                 if mode_m1 == -1
                   last_switch = tempo;
                   num_switch = num_switch + 1;
                 end
            else
                mode = -1;
                if mode_m1 == 1
                   last_switch = tempo;
                   num_switch = num_switch + 1;
                end
            end
        elseif de <= 0 && e >= 0
            % second quadrante
            if de >= -Mde && e <= Me
                 mode = 1;
                 if mode_m1 == -1
                   last_switch = tempo;
                   num_switch = num_switch + 1;
                 end
            else
                mode = -1;
                if mode_m1 == 1
                   last_switch = tempo;
                   num_switch = num_switch + 1;
                end
            end
        elseif de >= 0 && e <= 0
            % quarto quadrante
            if de <= Mde && e >= -Me
                 mode = 1;
                 if mode_m1 == -1
                   last_switch = tempo;
                   num_switch = num_switch + 1;
                 end
            else
                mode = -1;
                if mode_m1 == 1
                   last_switch = tempo;
                   num_switch = num_switch + 1;
                end
            end
        elseif de <= 0 && e <= 0
            % terzo quadrante
            if de >= -Mde && e >= -Me
                 mode = 1;
                 if mode_m1 == -1
                   last_switch = tempo;
                   num_switch = num_switch + 1;
                 end
            else
                mode = -1;
                if mode_m1 == 1
                   last_switch = tempo;
                   num_switch = num_switch + 1;
                end
            end
        end
    end
end


mode_m1 = mode;
ref_m1 = refs;
switches = num_switch;
last_sw = last_switch;
mode_n = mode;

end
